simulink model "MATLAB_Exercise_9"  (R2017b)
settings: Solver=VariableStepAuto  StartTime=0.0  StopTime=10.0  RelTol=1e-3
settings Model: Creator=chenjiasheng  LastModifiedBy=chenjiasheng

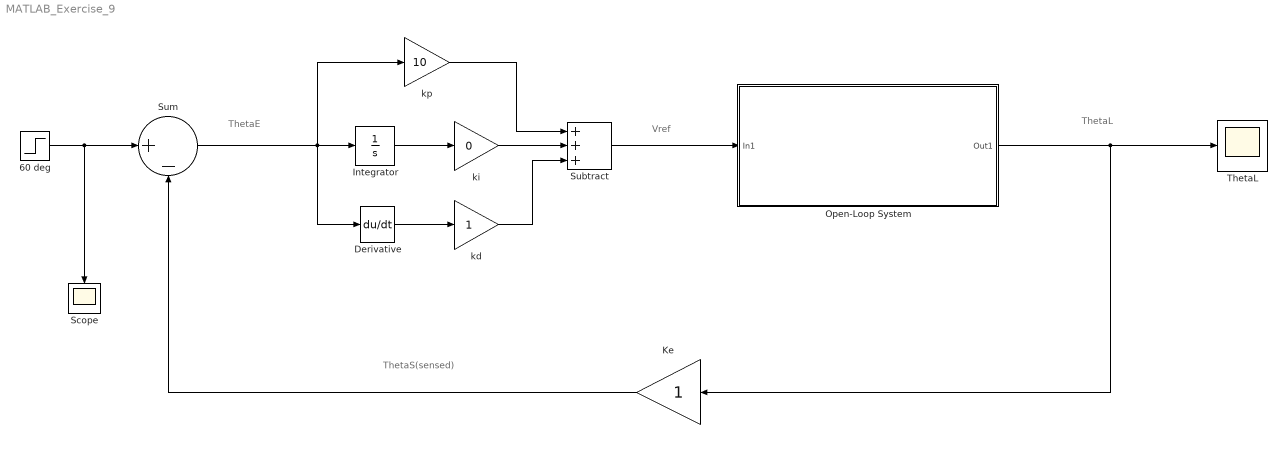
== system MATLAB_Exercise_9 ==
  note: Vref
  note: ThetaE
  note: ThetaS(sensed)
  note: ThetaL
  60 deg : Step  After=60  SampleTime=0
  Derivative : Derivative
  Integrator : Integrator
  Ke : Gain
  Open-Loop System : Subsystem
  Scope : Scope
  Subtract : Sum  Inputs=+++
  Sum : Sum  Inputs=|+-
  ThetaL : Scope
  kd : Gain
  ki : Gain  Gain=0
  kp : Gain  Gain=10
  wires:
  Open-Loop System/1(Out1) -> Ke/1, ThetaL/1
  Sum/1 -> Derivative/1, Integrator/1, kp/1
  kp/1 -> Subtract/1
  Subtract/1 -> Open-Loop System/1(In1)
  Ke/1 -> Sum/2
  60 deg/1 -> Sum/1, Scope/1
  Integrator/1 -> ki/1
  ki/1 -> Subtract/2
  kd/1 -> Subtract/3
  Derivative/1 -> kd/1

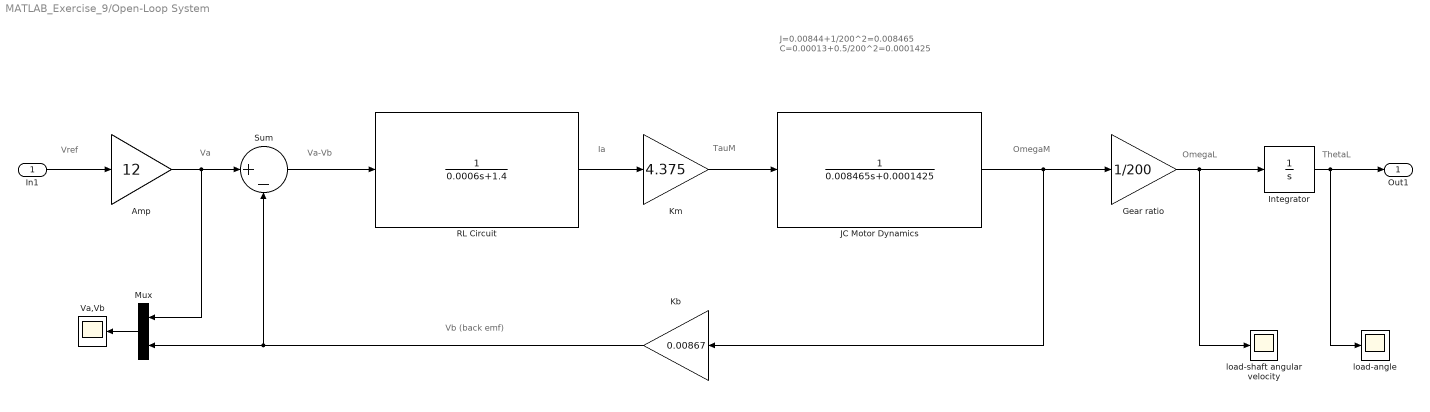
== system MATLAB_Exercise_9/Open-Loop System ==
  note: J=0.00844+1/200^2=0.008465
      | C=0.00013+0.5/200^2=0.0001425
  note: OmegaL
  note: OmegaM
  note: TauM
  note: Ia
  note: Va-Vb
  note: Va
  note: Vb (back emf)
  note: Vref
  note: ThetaL
  In1 : Inport
  " load-shaft angular velocity" : Scope
  Amp : Gain  Gain=12
  Gear ratio : Gain  Gain=1/200
  Integrator : Integrator
  JC Motor Dynamics : TransferFcn  Denominator=[0.008465 0.0001425]
  Kb : Gain  Gain=0.00867
  Km : Gain  Gain=4.375
  Mux : Mux  Inputs=2
  RL Circuit : TransferFcn  Denominator=[0.0006 1.4]
  Sum : Sum  Inputs=|+-
  Va,Vb : Scope
  load-angle : Scope
  Out1 : Outport
  wires:
  RL Circuit/1 -> Km/1
  Amp/1 -> Sum/1, Mux/1
  Sum/1 -> RL Circuit/1
  Km/1 -> JC Motor Dynamics/1
  JC Motor Dynamics/1 -> Kb/1, Gear ratio/1
  Kb/1 -> Mux/2, Sum/2
  Gear ratio/1 -> " load-shaft angular velocity"/1, Integrator/1
  In1/1 -> Amp/1
  Integrator/1 -> load-angle/1, Out1/1
  Mux/1 -> Va,Vb/1
